simulink model "Ex1sim"  (R2024b)
settings: Solver=VariableStepAuto  StartTime=0.0  StopTime=10.0  RelTol=1e-5
values from neighbouring files (symbols this model uses):
  Kd = Kp*Td    [Ex1.m]
  Ki = Kp/Ti    [Ex1.m]
  Kp = delta_K*cos(delta_phi)    [Ex1.m]
  kw = 1/(t_s/5)    [Ex1.m]
undefined symbols (not defined in the file or in its folder): tl
settings Model: Creator=bmm1  LastModifiedBy=bmm1

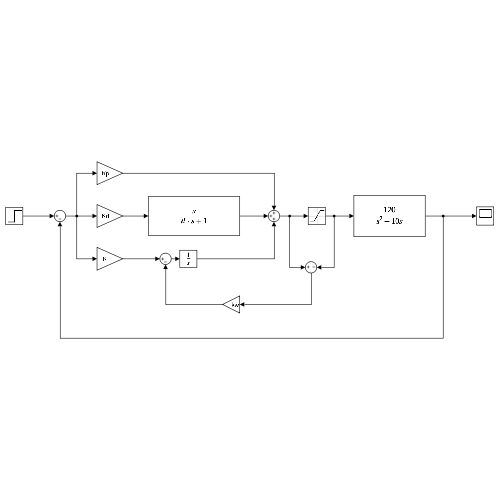
[thumbnail: Simulink's stored preview of the top-level diagram]
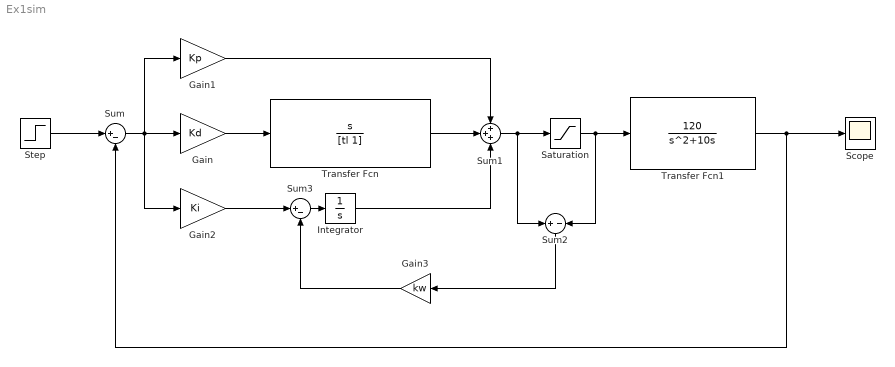
== system Ex1sim ==
  Gain : Gain  Gain=Kd
  Gain1 : Gain  Gain=Kp
  Gain2 : Gain  Gain=Ki
  Gain3 : Gain  Gain=kw
  Integrator : Integrator
  Saturation : Saturate  UpperLimit=10  LowerLimit=-10
  Scope : Scope
  Step : Step  After=120  SampleTime=0
  Sum : Sum  Inputs=|+-
  Sum1 : Sum  Inputs=+++
  Sum2 : Sum  Inputs=+|-
  Sum3 : Sum  Inputs=|+-
  Transfer Fcn : TransferFcn  Numerator=[1 0]  Denominator=[tl 1]
  Transfer Fcn1 : TransferFcn  Numerator=[120]  Denominator=[1 10 0]
  wires:
  Step/1 -> Sum/1
  Sum/1 -> Gain1/1, Gain2/1, Gain/1
  Gain/1 -> Transfer Fcn/1
  Integrator/1 -> Sum1/3
  Transfer Fcn/1 -> Sum1/2
  Gain1/1 -> Sum1/1
  Sum1/1 -> Sum2/1, Saturation/1
  Saturation/1 -> Sum2/2, Transfer Fcn1/1
  Sum2/1 -> Gain3/1
  Gain2/1 -> Sum3/1
  Sum3/1 -> Integrator/1
  Gain3/1 -> Sum3/2
  Transfer Fcn1/1 -> Sum/2, Scope/1
